simulink model "power_BuckConverter"  (R2021b)
settings: Solver=VariableStepAuto  StartTime=0.0  StopTime=0.008  MaxStep=1e-4  RelTol=1e-4  EnableMultiTasking=on
libraries: spsSeriesRLCBranchLib x3, spsDiodeLib x1, spsMosfetLib x1, spsPWMGeneratorDCDCLib x1, spsDCVoltageSourceLib x1, spsVoltageMeasurementLib x1, spspowerguiLib x1
settings Model: Creator=The MathWorks, Inc.  LastModifiedBy=caccolillo
settings SolverCC: AlgebraicLoopSolver=TrustRegion  SolverResetMethod=Robust
settings DataIOCC: ReturnWorkspaceOutputs=off
settings OptimizationCC: EfficientFloat2IntCast=on  LifeSpan=inf
settings DebuggingCC: UniqueDataStoreMsg=error  StrictBusMsg=ErrorOnBusTreatedAsVector  SFUnexpectedBacktrackingDiag=warning  SFNoUnconditionalDefaultTransitionDiag=warning  SFExecutionAtInitializationDiag=none  SFMachineParentedDataDiag=warning  ArithmeticOperatorsInVariantConditions=warning
settings SFSimCC: SimUseLocalCustomCode=off  CustomCodeUndefinedFunction=UseInterfaceOnly
settings RTWCC: RTWUseLocalCustomCode=off
settings CodeAppCC: StateflowObjectComments=on
settings GRTTargetCC: TargetLangStandard=C89/C90 (ANSI)
settings ConfigComp: CovMetricSettings=dw  CovSaveCumulativeToWorkspaceVar=on  CovSaveSingleToWorkspaceVar=on  CovExternalEMLEnable=off
settings SimscapeCC: SimscapeNormalizeSystem=off  SimscapeNominalValues={1, 'bar'; 1, 'cm^3/s'; 1, 'bar*kg/s'; 1, 'kJ/kg'; 1, 'kW'; }

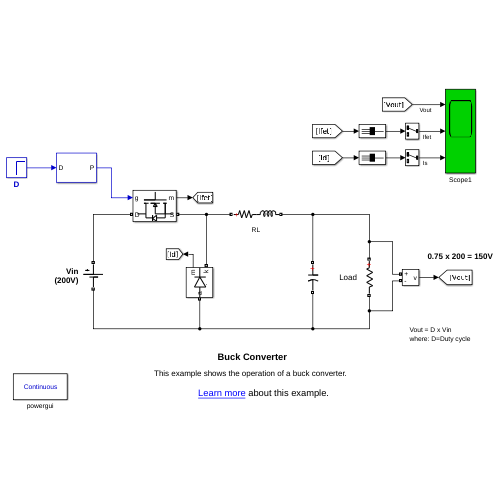
[thumbnail: Simulink's stored preview of the top-level diagram]
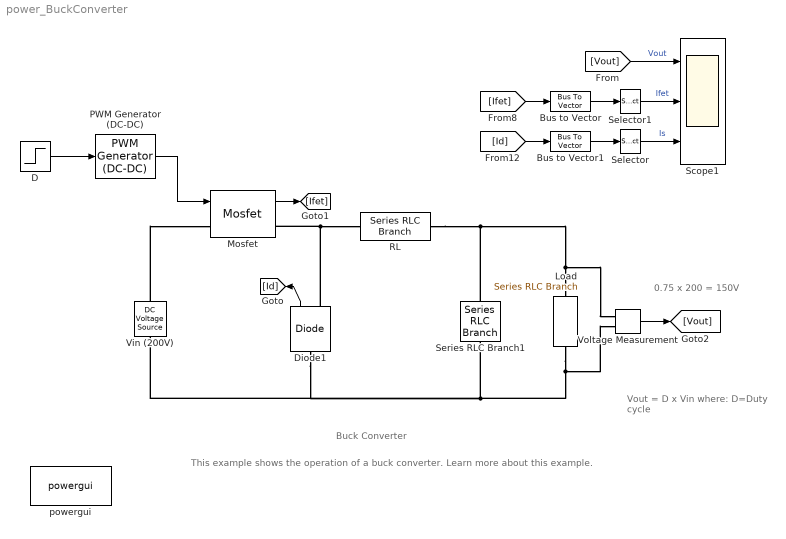
== system power_BuckConverter ==
  note: Vout = D x Vin
      | where: D=Duty cycle
  note: 0.75 x 200 = 150V
  note: This example shows the operation of a buck converter.
      |
      | Learn more about this example.
  note: Buck Converter
  Bus to Vector : BusToVector
  Bus to Vector1 : BusToVector
  D : Step  Time=0.0035  Before=0.5  After=0.75  SampleTime=0
  Diode1 : spsDiodeLib/Diode  Ron=1e-3  Lon=0  Vf=0  IC=0  UseSnubber=off  Rs=inf  Cs=inf  Measurements=on
  Load : spsSeriesRLCBranchLib/Series RLC Branch  LConnTagsString=__new0  RConnTagsString=__new0  BranchType=R  Resistance=10  Inductance=200e-6  SetiL0=off  InitialCurrent=0  Capacitance=400e-6  Setx0=off  InitialVoltage=0  Measurements=None
  Mosfet : spsMosfetLib/Mosfet  Ron=1e-3  Lon=0  Rd=1e-3  Vfd=0  IC=0  Rs=inf  Cs=inf  Measurements=on
  PWM Generator (DC-DC) : spsPWMGeneratorDCDCLib/PWM Generator (DC-DC)  Fsw=10e3  Ts=0
  RL : spsSeriesRLCBranchLib/Series RLC Branch  LConnTagsString=__new0  RConnTagsString=__new0  BranchType=RL  Resistance=0.02  Inductance=3e-3  SetiL0=off  InitialCurrent=0  Capacitance=1e-6  Setx0=off  InitialVoltage=0  Measurements=None
  Scope1 : Scope  NumInputPorts=3
  Selector : Selector  InputPortWidth=2  IndexOptions=Index vector (dialog)  Indices=1  OutputSizes=1
  Selector1 : Selector  InputPortWidth=2  IndexOptions=Index vector (dialog)  Indices=1  OutputSizes=1
  Series RLC Branch1 : spsSeriesRLCBranchLib/Series RLC Branch  LConnTagsString=__new0  RConnTagsString=__new0  BranchType=C  Resistance=1e-4  Inductance=200e-6  SetiL0=off  InitialCurrent=0  Capacitance=30e-6  Setx0=off  InitialVoltage=150  Measurements=None
  Vin (200V) : spsDCVoltageSourceLib/DC Voltage Source  Amplitude=200  Measurements=None
  Voltage Measurement : spsVoltageMeasurementLib/Voltage Measurement  PhasorSimulation=off  OutputType=Complex  PSBequivalent=0
  powergui : spspowerguiLib/powergui  Priority=1  SimulationMode=Continuous  SampleTime=50e-6  frequency=60  Iterations=50  frequencyindice=0  Pbase=100e6  ErrMax=1e-4  UnitsV=kV  UnitsW=MW  buscounter=0  FunctionMessages=off  echomessages=off  EnableUseOfTLC=off  CurrentSourceSwitches=off  DisableSnubberDevices=off  DisableRonSwitches=off  DisableVfSwitches=off  DisplayEquations=off  AutomaticDiscreteSolvers=off  SolverType=Tustin/Backward Euler (TBE)  Interpol=off  ExternalGateDelay=off  methode=off  Ts=100  x0status=blocks  SPID=on  SwTol=0  HookPort=off  NonlinearTolerance=1e-4  nMaxIteration=100  ContinueOnMaxIteration=off  RestoreLinks=warning  ResistiveCurrentMeasurement=off  Frange=[0:2:500]  Ylog=off  Xlog=on  ShowGrid=off  save=off  variable=ZData  structure=0  ZoomFFT=off  StartTime=0.0  cycles=1  DisplayStyle=1  fundamental=60  FreqAxis=off  MaxFrequency=1000  frequencyindicesteady=1  RmsSteady=1  display=off
  wires:
  Diode1/1 -> [Id]
  Voltage Measurement/1 -> [Vout]
  [Ifet] -> Bus to Vector/1
  [Id] -> Bus to Vector1/1
  Mosfet/1 -> [Ifet]
  PWM Generator (DC-DC)/1 -> Mosfet/1
  Selector1/1 -> Scope1/2  "Ifet"
  Selector/1 -> Scope1/3  "Is"
  D/1 -> PWM Generator (DC-DC)/1
  [Vout] -> Scope1/1  "Vout"
  Bus to Vector/1 -> Selector1/1
  Bus to Vector1/1 -> Selector/1
  connections:
  Load/RConn1 -- Vin (200V)/LConn1 -- Diode1/LConn1 -- Series RLC Branch1/RConn1 -- Voltage Measurement/LConn2
  Series RLC Branch1/LConn1 -- Voltage Measurement/LConn1 -- Load/LConn1 -- RL/RConn1
  Vin (200V)/RConn1 -- Mosfet/LConn1
  Diode1/RConn1 -- RL/LConn1 -- Mosfet/RConn1
